simulink model "power_aircraft_distribution_mexido_2016_V6_comfiltro_export"  (R2015b)
settings: Solver=FixedStepAuto  StartTime=72.85  StopTime=73.9  MaxStep=0.01  RelTol=0.2e-4  AbsTol=0.2e-4
PreLoadFcn:
  | % -- Recommended Settings --
  | %
  | %  Simulink:
  | %      Solver: Ode23t
  | %      Relative tolerance = 1e-3
  | %       Max step size = 0.2
  | %
  | %  Powergui:
  |          Ts = 1e-07; % (discrete electrical model)
  | %
  | %  Control systems:
  |          Ts_control = 10*Ts; % (discrete control system)
  | %
  | % ----------------------------------
values from neighbouring files (symbols this model uses):
  D1 = k/M+A^2*beta/(V0*M)+beta*Ct*B/(V0*M)    (= 3003877.72556)    [EHA.m]
undefined symbols (not defined in the file or in its folder): C, Delta, L, sigbuilder_block
libraries: powerlib x79, dsparch4 x12, simulink x6, sps_avr x1, powerlib_meascontrol x1
(part 3 of 3)

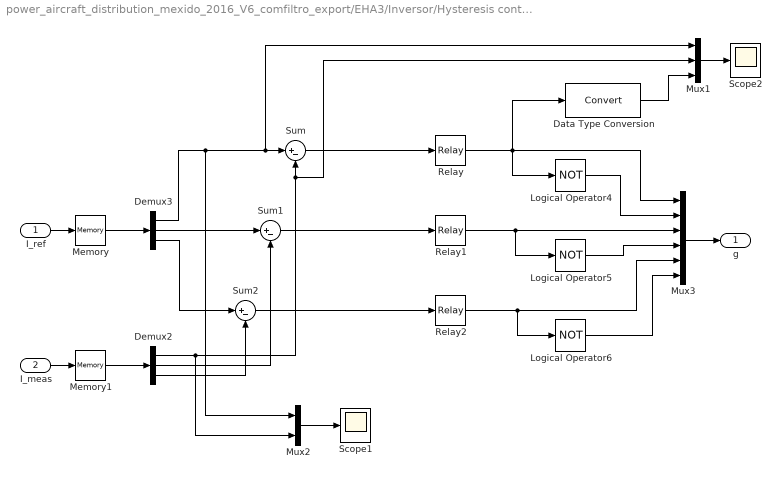
== system power_aircraft_distribution_mexido_2016_V6_comfiltro_export/EHA3/Inversor/Hysteresis controller ==
  I_ref : Inport
  I_meas : Inport  Port=2
  Data Type Conversion : DataTypeConversion
  Demux2 : Demux  Outputs=3
  Demux3 : Demux  Outputs=3
  Logical Operator4 : Logic  Operator=NOT  AllPortsSameDT=off  OutDataTypeStr=boolean
  Logical Operator5 : Logic  Operator=NOT  AllPortsSameDT=off  OutDataTypeStr=boolean
  Logical Operator6 : Logic  Operator=NOT  AllPortsSameDT=off  OutDataTypeStr=boolean
  Memory : Memory
  Memory1 : Memory
  Mux1 : Mux  Inputs=3
  Mux2 : Mux  Inputs=2
  Mux3 : Mux  Inputs=6
  Relay : Relay  OnSwitchValue=0.05  OffSwitchValue=-0.05  OutDataTypeStr=Inherit: Inherit via back propagation
  Relay1 : Relay  OnSwitchValue=0.05  OffSwitchValue=-0.05  OutDataTypeStr=Inherit: Inherit via back propagation
  Relay2 : Relay  OnSwitchValue=0.05  OffSwitchValue=-0.05  OutDataTypeStr=Inherit: Inherit via back propagation
  Scope1 : Scope
  Scope2 : Scope
  Sum : Sum  Inputs=|+-
  Sum1 : Sum  Inputs=|+-
  Sum2 : Sum  Inputs=|+-
  g : Outport
  wires:
  I_ref/1 -> Memory/1
  I_meas/1 -> Memory1/1
  Relay1/1 -> Logical Operator5/1, Mux3/3
  Demux3/1 -> Mux1/1, Sum/1, Mux2/1
  Logical Operator4/1 -> Mux3/2
  Logical Operator5/1 -> Mux3/4
  Logical Operator6/1 -> Mux3/6
  Mux3/1 -> g/1
  Demux2/1 -> Mux2/2, Mux1/2, Sum/2
  Memory/1 -> Demux3/1
  Memory1/1 -> Demux2/1
  Mux2/1 -> Scope1/1
  Relay/1 -> Data Type Conversion/1, Mux3/1, Logical Operator4/1
  Demux3/2 -> Sum1/1
  Demux2/2 -> Sum1/2
  Demux3/3 -> Sum2/1
  Demux2/3 -> Sum2/2
  Relay2/1 -> Mux3/5, Logical Operator6/1
  Mux1/1 -> Scope2/1
  Data Type Conversion/1 -> Mux1/3
  Sum/1 -> Relay/1
  Sum1/1 -> Relay1/1
  Sum2/1 -> Relay2/1

== system power_aircraft_distribution_mexido_2016_V6_comfiltro_export/EHA3/Inversor/PI controller ==
  Vdc : Inport
  LPF : dsparch4/Analog Filter Design  method=Butterworth  filttype=Lowpass  N=5  Wlo=2*pi*200  Whi=80  Rp=2  Rs=40
  PID Controller : simulink/Continuous/PID Controller  Controller=PI  TimeDomain=Continuous-time  SampleTime=-1  IntegratorMethod=Forward Euler  FilterMethod=Forward Euler  Form=Parallel  UseFilter=on  ControllerParametersSource=internal  P=5  I=7  D=0  N=100  InitialConditionSource=internal  InitialConditionForIntegrator=0  InitialConditionForFilter=0  ExternalReset=none  LimitOutput=off  UpperSaturationLimit=inf  LowerSaturationLimit=-inf  LinearizeAsGain=on  AntiWindupMode=none  Kb=1  TrackingMode=off  Kt=1  PParamMin=[]  PParamMax=[]  IParamMin=[]  IParamMax=[]  DParamMin=[]  DParamMax=[]  NParamMin=[]  NParamMax=[]  KbParamMin=[]  KbParamMax=[]  KtParamMin=[]  KtParamMax=[]  POutMin=[]  POutMax=[]  IOutMin=[]  IOutMax=[]  DOutMin=[]  DOutMax=[]  NOutMin=[]  NOutMax=[]  KbOutMin=[]  KbOutMax=[]  KtOutMin=[]  KtOutMax=[]  IntegratorOutMin=[]  IntegratorOutMax=[]  FilterOutMin=[]  FilterOutMax=[]  SumOutMin=[]  SumOutMax=[]  SumI1OutMin=[]  SumI1OutMax=[]  SumI2OutMin=[]  SumI2OutMax=[]  SumI3OutMin=[]  SumI3OutMax=[]  SumDOutMin=[]  SumDOutMax=[]  SaturationOutMin=[]  SaturationOutMax=[]  IntegratorContinuousStateAttributes=''  IntegratorStateMustResolveToSignalObject=off  IntegratorRTWStateStorageClass=Auto  FilterContinuousStateAttributes=''  FilterStateMustResolveToSignalObject=off  FilterRTWStateStorageClass=Auto  DifferentiatorICPrevScaledInput=0  DifferentiatorOutMin=[]  DifferentiatorOutMax=[]
  Scope : Scope  NumInputPorts=2
  Signal Builder1 : Subsystem  Tag=STV Subsys  LoadFcn=sigbuilder_block('load');  StartFcn=sigbuilder_block('start');  StopFcn=sigbuilder_block('stop');  ClipboardFcn=sigbuilder_block('clipboard');  mask(Sigbuilder block){}
      mask help: Simulink:masks:SigbuilderBlock_MD
      mask init:
      | if ~strcmp(get_param(bdroot(gcbh),'SimulationStatus'),'stopped') tuvar = sigbuilder_block('maskInit'); end
      settings: CopyFcn=sigbuilder_block('copy');  DeleteFcn=sigbuilder_block('delete');  ModelCloseFcn=sigbuilder_block('modelClose');  PreSaveFcn=sigbuilder_block('preSave');  PauseFcn=sigbuilder_block('pause');  ContinueFcn=sigbuilder_block('continue');  NameChangeFcn=sigbuilder_block('namechange');  OpenFcn=sigbuilder_block('open',[437.6 199.2 550.4 400 ]);  CloseFcn=sigbuilder_block('close');
      mask Display: plot(0, 0, 100, 100,[2, 2, 32, 32, 2], [68, 8, 8, 68, 68],[32, 2], [38, 38], [32, 19, 2],[53, 60, 44], [32, 17, 17, 2],[16, 16, 31, 31]);txt = getActiveGroup(gcbh);text(2, 100, txt,'verticalAlignment', 'top');
  Sum : Sum  Inputs=|-+
  Ploss : Outport
  wires:
  Vdc/1 -> Scope/1, Sum/1  "Vdc3"
  Sum/1 -> Scope/2, LPF/1  "Vdc3-step"
  Signal Builder1/1(Signal 1) -> Sum/2
  PID Controller/1 -> Ploss/1
  LPF/1 -> PID Controller/1

== system power_aircraft_distribution_mexido_2016_V6_comfiltro_export/EHA1/Inversor/PI controller/Signal Builder1 ==
  Demux : Demux  Tag=STV Demux  Outputs=1
  FromWs : FromWorkspace  Tag=STV FromWs  VariableName=tuvar  SampleTime=0
      SigBuilderData=|
      | common.afterFinalStr = 'Extrapolate'
      | common.sampleTime = 0
      | dataSet.timeRange = [0 74]
      | dataSet.name = 'Group 1'
      | sbobj.Groups.Name = 'Group 1'
      | sbobj.Groups.Signals.Name = 'Signal 1'
      | sbobj.Groups.Signals.XData = [0 72.66 72.66 74]
      | sbobj.Groups.Signals.YData = [0 0 560 560]
      | sbobj.Groups.TimeRange = [0 74]
  Signal 1 : Outport  Tag=STV Outport
  wires:
  Demux/1 -> Signal 1/1
  FromWs/1 -> Demux/1

== system power_aircraft_distribution_mexido_2016_V6_comfiltro_export/EHA2/Inversor/PI controller/Signal Builder1 ==
  Demux : Demux  Tag=STV Demux  Outputs=1
  FromWs : FromWorkspace  Tag=STV FromWs  VariableName=tuvar  SampleTime=0
      SigBuilderData=|
      | common.afterFinalStr = 'Extrapolate'
      | common.sampleTime = 0
      | dataSet.timeRange = [0 74]
      | dataSet.name = 'Group 1'
      | sbobj.Groups.Name = 'Group 1'
      | sbobj.Groups.Signals.Name = 'Signal 1'
      | sbobj.Groups.Signals.XData = [0 72.66 72.66 74]
      | sbobj.Groups.Signals.YData = [0 0 560 560]
      | sbobj.Groups.TimeRange = [0 74]
  Signal 1 : Outport  Tag=STV Outport
  wires:
  Demux/1 -> Signal 1/1
  FromWs/1 -> Demux/1

== system power_aircraft_distribution_mexido_2016_V6_comfiltro_export/EHA3/Inversor/PI controller/Signal Builder1 ==
  Demux : Demux  Tag=STV Demux  Outputs=1
  FromWs : FromWorkspace  Tag=STV FromWs  VariableName=tuvar  SampleTime=0
      SigBuilderData=|
      | common.afterFinalStr = 'Extrapolate'
      | common.sampleTime = 0
      | dataSet.timeRange = [0 74]
      | dataSet.name = 'Group 1'
      | sbobj.Groups.Name = 'Group 1'
      | sbobj.Groups.Signals.Name = 'Signal 1'
      | sbobj.Groups.Signals.XData = [0 72.66 72.66 74]
      | sbobj.Groups.Signals.YData = [0 0 560 560]
      | sbobj.Groups.TimeRange = [0 74]
  Signal 1 : Outport  Tag=STV Outport
  wires:
  Demux/1 -> Signal 1/1
  FromWs/1 -> Demux/1
